simulink library "Window_Ventilation"  (Simulink 8.2)
settings: Solver=ode45  StartTime=0.0  StopTime=10.0  RelTol=1e-3
settings Model: Creator=lena.frank  LastModifiedBy=ralf.dott  CovSaveCumulativeToWorkspaceVar=on

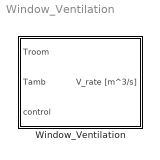
== system Window_Ventilation ==
  Window_Ventilation : Subsystem  mask(window ventilation){alpha=10, H=1, W=1}
      mask prompts: alpha "maximal opening angle (°)"; H "height of window (m)"; W "width of window (m)"
      mask help: Simulates the free driven ventilation through a window with an opening angle of [0,1]* max. angle. Valid for angles between 8° and 180°. Output is the VOLUME FLOW RATE in m^3/s. Calculation based on the approach from Weber.
      mask Help: web(fullfile(path_carnot('help'),'Window_Ventilation.html'),'-helpbrowser')
      mask Display: plot(0,10,90,80,[20 70 70 20 20],[20 20 70 70 20],[20 70 80 30 20],[20 20 65 65 20])

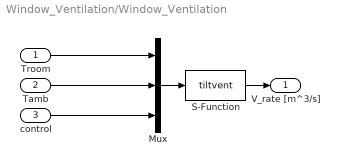
== system Window_Ventilation/Window_Ventilation ==
  Troom : Inport
  Tamb : Inport  Port=2
  control : Inport  Port=3
  Mux : Mux  Inputs=3
  S-Function : S-Function  FunctionName=tiltvent  Parameters=alpha, H, W  SFunctionDeploymentMode=off  EnableBusSupport=off
  V_rate [m^3/s] : Outport
  wires:
  Troom/1 -> Mux/1
  Mux/1 -> S-Function/1
  S-Function/1 -> V_rate [m^3/s]/1
  control/1 -> Mux/3
  Tamb/1 -> Mux/2
